simulink model "lp_01"  (R2019a)
settings: Solver=VariableStepAuto  StartTime=0.0  StopTime=0.5  RelTol=1e-3
libraries: dspsrcs4 x2, dsparch4 x1
settings Model: Creator=Zhiguo  LastModifiedBy=Zhiguo

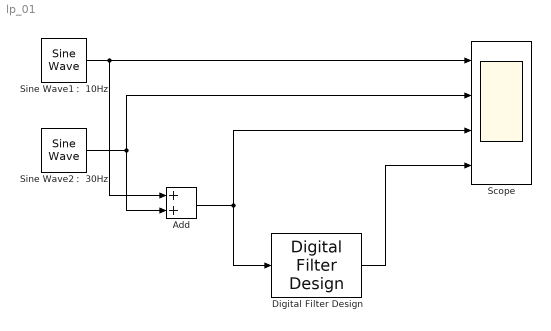
== system lp_01 ==
  Add : Sum
  Digital Filter Design : dsparch4/Digital Filter Design  mwdsp_browser_bugfix_var=off
  Scope : Scope  NumInputPorts=4
  Sine Wave1： 10Hz : dspsrcs4/Sine Wave  Amplitude=1  Frequency=5  Phase=0  SampleMode=Discrete  OutComplex=Real  CompMethod=Trigonometric fcn  TableSize=Speed  SampleTime=1/1000  SamplesPerFrame=1  ResetState=Restart at time zero  OutputFrames=off  dataType=double  wordLen=16  udDataType=sfix(16)  fracBitsMode=Best precision  numFracBits=15  OutDataTypeStr=double  LastOutDataTypeStr=double
  Sine Wave2： 30Hz : dspsrcs4/Sine Wave  Amplitude=1  Frequency=80  Phase=0  SampleMode=Discrete  OutComplex=Real  CompMethod=Trigonometric fcn  TableSize=Speed  SampleTime=1/1000  SamplesPerFrame=1  ResetState=Restart at time zero  OutputFrames=off  dataType=double  wordLen=16  udDataType=sfix(16)  fracBitsMode=Best precision  numFracBits=15  OutDataTypeStr=double  LastOutDataTypeStr=double
  wires:
  Sine Wave1： 10Hz/1 -> Add/1, Scope/1
  Sine Wave2： 30Hz/1 -> Add/2, Scope/2
  Add/1 -> Digital Filter Design/1, Scope/3
  Digital Filter Design/1 -> Scope/4
